simulink library "magnetic_torque"  (R2021b)
settings: Solver=VariableStepAuto  StartTime=0.0  StopTime=10.0  RelTol=1e-3
values from neighbouring files (symbols this model uses):
  init_mjd2000 = 0    [initial_conditions.m]    (also in magnetic_init.m)
  t0 = 0    [initial_conditions.m]    (also in magnetic_init.m)
  theta_g0 = 0    [initial_conditions.m]    (also in magnetic_init.m)
  we = 7.2916e-05    [initial_conditions.m]    (also in magnetic_init.m)
libraries: vrlib x1, matrix_library x1
settings Model: Creator=white  LastModifiedBy=white

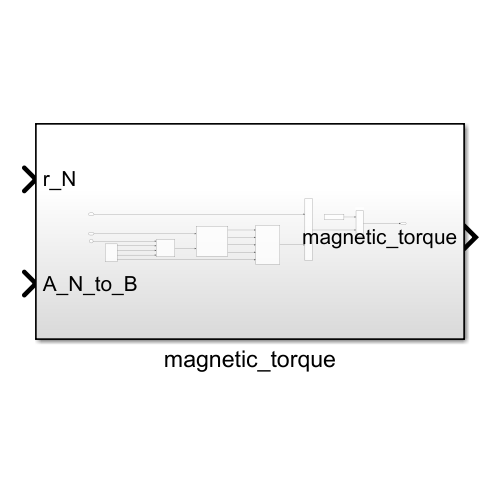
[thumbnail: Simulink's stored preview of the top-level diagram]
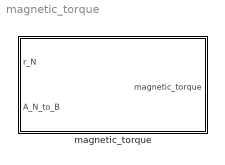
== system magnetic_torque ==
  magnetic_torque : Subsystem

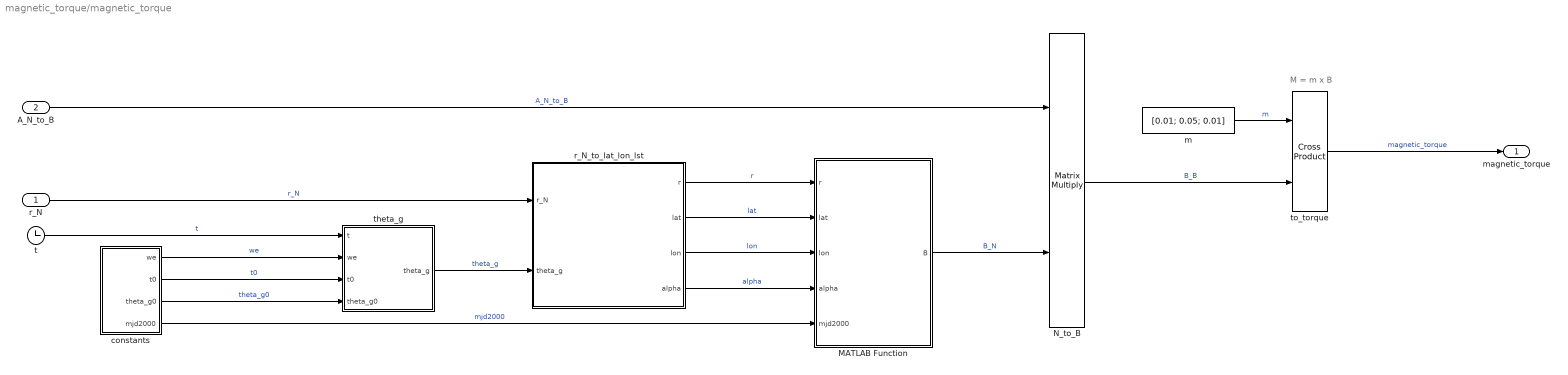
== system magnetic_torque/magnetic_torque ==
  note: M = m x B
  r_N : Inport
  A_N_to_B : Inport  Port=2
  MATLAB Function : MATLAB Function  TreatAsAtomicUnit=on
  N_to_B : Product  Multiplication=Matrix(*)
  constants : Subsystem
  m : Constant  Value=[0.01; 0.05; 0.01]
  r_N_to_lat_lon_lst : Subsystem
  t : Clock
  theta_g : Subsystem
  to_torque : matrix_library/Cross Product
      settings: SourceProductBaseCode=SL
  magnetic_torque : Outport
  wires:
  r_N/1 -> r_N_to_lat_lon_lst/1(r_N)  "r_N"
  r_N_to_lat_lon_lst/2(lat) -> MATLAB Function/2(lat)  "lat"
  r_N_to_lat_lon_lst/3(lon) -> MATLAB Function/3(lon)  "lon"
  A_N_to_B/1 -> N_to_B/1  "A_N_to_B"
  MATLAB Function/1(B) -> N_to_B/2  "B_N"
  N_to_B/1 -> to_torque/2  "B_B"
  to_torque/1 -> magnetic_torque/1  "magnetic_torque"
  m/1 -> to_torque/1  "m"
  r_N_to_lat_lon_lst/1(r) -> MATLAB Function/1(r)  "r"
  r_N_to_lat_lon_lst/4(alpha) -> MATLAB Function/4(alpha)  "alpha"
  theta_g/1(theta_g) -> r_N_to_lat_lon_lst/2(theta_g)  "theta_g"
  t/1 -> theta_g/1(t)  "t"
  constants/3(theta_g0) -> theta_g/4(theta_g0)  "theta_g0"
  constants/2(t0) -> theta_g/3(t0)  "t0"
  constants/1(we) -> theta_g/2(we)  "we"
  constants/4(mjd2000) -> MATLAB Function/5(mjd2000)  "mjd2000"

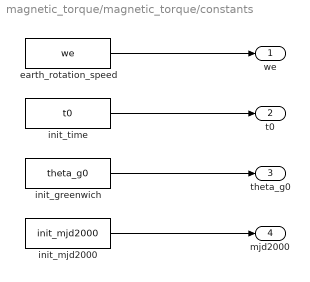
== system magnetic_torque/magnetic_torque/constants ==
  earth_rotation_speed : Constant  Value=we
  init_greenwich : Constant  Value=theta_g0
  init_mjd2000 : Constant  Value=init_mjd2000
  init_time : Constant  Value=t0
  we : Outport
  t0 : Outport  Port=2
  theta_g0 : Outport  Port=3
  mjd2000 : Outport  Port=4
  wires:
  init_mjd2000/1 -> mjd2000/1
  init_greenwich/1 -> theta_g0/1
  init_time/1 -> t0/1
  earth_rotation_speed/1 -> we/1

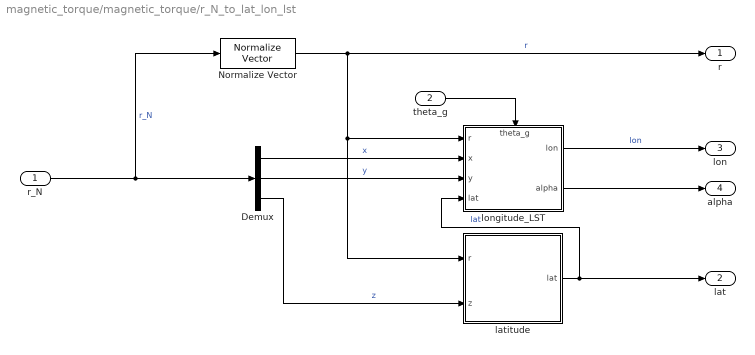
== system magnetic_torque/magnetic_torque/r_N_to_lat_lon_lst ==
  r_N : Inport
  theta_g : Inport  Port=2
  Demux : Demux  Outputs=3
  Normalize Vector : vrlib/Utilities/Normalize Vector  maxzero=0
  latitude : Subsystem
  longitude_LST : Subsystem
      settings: PortSchema="{\"entries\":[{\"content\":{\"sides\":[{\"content\":{\"connectorIds\":[\"In1\",\"In2\",\"In3\",\"In4\"]},\"type\":\"ConnectorPlacement.EquallySpacedRectSide\",\"uuid\":\"b197dfa4-c230-4803-a0b3-2d3c44e10a73\"},{\"content\":{\"connectorIds\":[\"Out1\",\"Out2\"],\"side\":\"RIGHT\"},\"type\":\"ConnectorPlacement.EquallySpacedRectSide\",\"uuid\":\"0aaebfc3-1b92-4483-8724-e78c586dcfa0\"},{\"content\":{\"connectorIds\":[\"In5\"],\"side\":\"TOP\"},\"type\":\"ConnectorPlacement.EquallySpacedRectSide\",\"uuid\":\"07c76325-0830-48dd-a056-b0076ab4a89f\"}]},\"type\":\"ConnectorPlacement.EquallySpacedConnector\",\"uuid\":\"374bbd02-45c5-4bda-9379-dc8e2163807b\"}],\"packageUris\":[\"http://schema.mathworks.com/mf0/Connector/R2020b\"],\"version\":\"1.0\"}"
  r : Outport
  lat : Outport  Port=2
  lon : Outport  Port=3
  alpha : Outport  Port=4
  wires:
  r_N/1 -> Demux/1, Normalize Vector/1  "r_N"
  Demux/1 -> longitude_LST/2(x)  "x"
  Normalize Vector/1 -> latitude/1(r), longitude_LST/1(r), r/1  "r"
  Demux/3 -> latitude/2(z)  "z"
  latitude/1(lat) -> longitude_LST/4(lat), lat/1  "lat"
  Demux/2 -> longitude_LST/3(y)  "y"
  longitude_LST/1(lon) -> lon/1  "lon"
  longitude_LST/2(alpha) -> alpha/1
  theta_g/1 -> longitude_LST/5(theta_g)

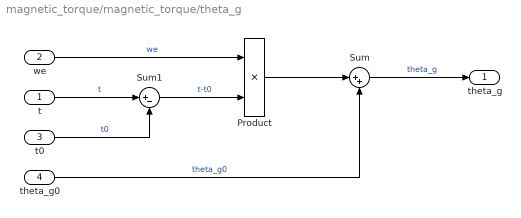
== system magnetic_torque/magnetic_torque/theta_g ==
  t : Inport
  we : Inport  Port=2
  t0 : Inport  Port=3
  theta_g0 : Inport  Port=4
  Product : Product
  Sum : Sum  Inputs=|++
  Sum1 : Sum  Inputs=|+-
  theta_g : Outport
  wires:
  t0/1 -> Sum1/2  "t0"
  Sum1/1 -> Product/2  "t-t0"
  t/1 -> Sum1/1  "t"
  theta_g0/1 -> Sum/2  "theta_g0"
  we/1 -> Product/1  "we"
  Product/1 -> Sum/1
  Sum/1 -> theta_g/1  "theta_g"

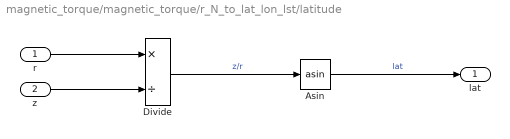
== system magnetic_torque/magnetic_torque/r_N_to_lat_lon_lst/latitude ==
  r : Inport
  z : Inport  Port=2
  Asin : Trigonometry  Operator=asin
  Divide : Product  Inputs=*/
  lat : Outport
  wires:
  z/1 -> Divide/2
  Divide/1 -> Asin/1  "z/r"
  r/1 -> Divide/1
  Asin/1 -> lat/1  "lat"

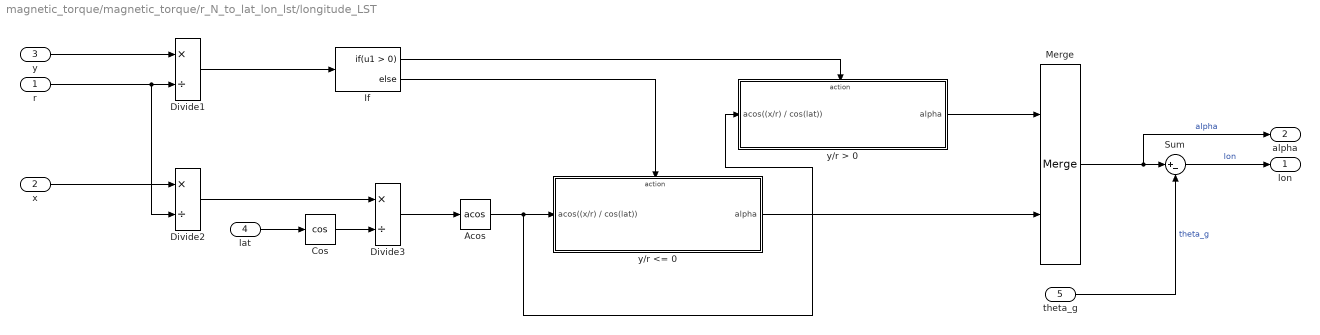
== system magnetic_torque/magnetic_torque/r_N_to_lat_lon_lst/longitude_LST ==
  r : Inport
  x : Inport  Port=2
  y : Inport  Port=3
  lat : Inport  Port=4
  theta_g : Inport  Port=5
  Acos : Trigonometry  Operator=acos
  Cos : Trigonometry  Operator=cos
  Divide1 : Product  Inputs=*/
  Divide2 : Product  Inputs=*/
  Divide3 : Product  Inputs=*/
  If : If
  Merge : Merge
  Sum : Sum  Inputs=|+-
  y/r <= 0 : Subsystem  TreatAsAtomicUnit=on
  "y/r > 0 " : Subsystem  TreatAsAtomicUnit=on
  lon : Outport
  alpha : Outport  Port=2
  wires:
  Divide1/1 -> If/1
  r/1 -> Divide1/2, Divide2/2
  y/1 -> Divide1/1
  If/1 -> "y/r > 0 "/Action
  If/2 -> y/r <= 0/Action
  "y/r > 0 "/1(alpha) -> Merge/1
  y/r <= 0/1(alpha) -> Merge/2
  Merge/1 -> alpha/1, Sum/1  "alpha"
  theta_g/1 -> Sum/2  "theta_g"
  Sum/1 -> lon/1  "lon"
  x/1 -> Divide2/1
  Divide2/1 -> Divide3/1
  Divide3/1 -> Acos/1
  Cos/1 -> Divide3/2
  lat/1 -> Cos/1
  Acos/1 -> "y/r > 0 "/1(acos((x/r) / cos(lat))), y/r <= 0/1(acos((x/r) / cos(lat)))

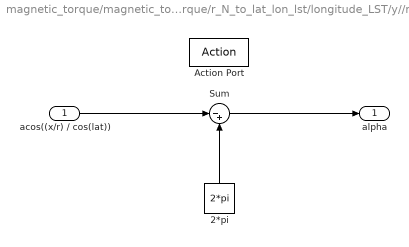
== system magnetic_torque/magnetic_torque/r_N_to_lat_lon_lst/longitude_LST/y//r <= 0 ==
  acos((x/r) / cos(lat)) : Inport
  Action Port : ActionPort  ActionPortLabel=else
  2*pi : Constant  Value=2*pi
  Sum : Sum  Inputs=|-+
  alpha : Outport
  wires:
  acos((x/r) / cos(lat))/1 -> Sum/1
  2*pi/1 -> Sum/2
  Sum/1 -> alpha/1

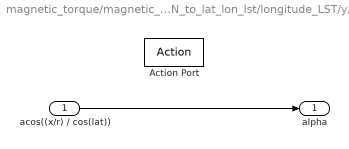
== system magnetic_torque/magnetic_torque/r_N_to_lat_lon_lst/longitude_LST/y//r > 0  ==
  acos((x/r) / cos(lat)) : Inport
  Action Port : ActionPort  ActionPortLabel=if(u1 > 0)
  alpha : Outport
  wires:
  acos((x/r) / cos(lat))/1 -> alpha/1

== matlab function magnetic_torque/MATLAB Function ==
  data: r input; B output; lat input; lon input; alpha input; mjd2000 input
function B = magnet(r, lat, lon, alpha, mjd2000)
    % Inputs
    % r Geocentric radius
    % lat Latitude measured in degrees positive from equator
    % lon Longitude measured in degrees positive east from Greenwich
    % alpha Local sidereal time of location (in degrees)
    % mjd2000 Decimal days since January 1, 2000
    %
    % Outputs
    % Bx B in x-direction | Magnetic field strength (B)
    % By B in y-direction | in geocentric inertial coordinates
    % Bz B in z-direction |

    % Checks to see if located at either pole to avoid singularities
    if (lat > -0.00000001 && lat < 0.00000001)
        lat = 0.00000001;
    elseif(lat < 180.00000001 && lat > 179.99999999)
        lat = 179.99999999;
    end

    % The angles must be converted from degrees into radians
    lat = (90 - lat) * pi/180;  % co-latitude
    lon = lon * pi/180;
    a = 6371.2; % Reference radius used in IGRF

    % This section of the code simply reads in the g and h Schmidt
    % quasi-normalized coefficients
    igrfSg = fopen('igrfSg.txt');
    igrfSh = fopen('igrfSh.txt');
    [gn, gm, gvali, gsvi] = textscan(igrfSg, '%f %f %f %f');
    [hn, hm, hvali, hsvi] = textscan(igrfSh, '%f %f %f %f');

    N = max(gn);
    g = zeros(N, N+1);
    h = zeros(N, N+1);

    for x=1:length(gn)
        g(gn(x), gm(x)+1) = gvali(x) + gsvi(x) * mjd2000/365;
        h(hn(x), hm(x)+1) = hvali(x) + hsvi(x) * mjd2000/365;
    end

    % Initialize each of the variables
    % Br B in the radial driection
    % Bt B in the theta direction
    % Bp B in the phi direction
    % P The associated Legendre polynomial evaluated at cos(theta)
    % The nomenclature for the recursive values generally follows
    % the form P10 = P(n-1,m-0)
    % dP The partial derivative of P with respect to theta
    Br = 0; Bt = 0; Bp = 0;
    P11 = 1; P10 = P11;
    dP11 = 0; dP10 = dP11;

    for m = 0:N
        for n = 1:N
            if m <= n
                % Calculate Legendre polynomials and derivatives recursively
                if n == m
                    P2 = sin(lat)*P11;
                    dP2 = sin(lat)*dP11 + cos(lat)*P11;
                    P11 = P2; P10 = P11; P20 = 0;
                    dP11 = dP2; dP10 = dP11; dP20 = 0;
                elseif n == 1
                    P2 = cos(lat)*P10;
                    dP2 = cos(lat)*dP10 - sin(lat)*P10;
                    P20 = P10; P10 = P2;
                    dP20 = dP10; dP10 = dP2;
                else
                    K = ((n-1)^2-m^2) / ((2*n-1)*(2*n-3));
                    P2 = cos(lat)*P10 - K*P20;
                    dP2 = cos(lat)*dP10 - sin(lat)*P10 - K*dP20;
                    P20 = P10; P10 = P2;
                    dP20 = dP10; dP10 = dP2;
                end

                % Calculate Br, Bt, and Bp
                Br = Br + (a/r)^(n+2)*(n+1)*...
                ((g(n,m+1)*cos(m*lon) + h(n,m+1)*sin(m*lon))*P2);

                Bt = Bt + (a/r)^(n+2)*...
                ((g(n,m+1)*cos(m*lon) + h(n,m+1)*sin(m*lon))*dP2);

                Bp = Bp + (a/r)^(n+2)*...
                (m*(-g(n,m+1)*sin(m*lon) + h(n,m+1)*cos(m*lon))* P2);
            end
        end
    end
    Bt = -Bt; Bp = -Bp/sin(lat);

    % Angle conversion to radians
    lat = lat * pi/180; alpha = alpha * pi/180;
    % Coordinate transformation
    Bx = (Br*cos(lat)+Bt*sin(lat))*cos(alpha) - Bp*sin(alpha);
    By = (Br*cos(lat)+Bt*sin(lat))*sin(alpha) + Bp*cos(alpha);
    Bz = (Br*sin(lat)+Bt*cos(lat));

    B = [Bx; By; Bz];
end
